simulink model "object_os"  (Simulink 8.7)
settings: Solver=ode45  StartTime=0.0  StopTime=3  FixedStep=0.01  RelTol=1e-3
settings Model: Creator=Andrew  LastModifiedBy=Dima
settings DataIOCC: ExternalInput=[a]  SignalLoggingSaveFormat=ModelDataLogs  SignalLogging=off  DSMLogging=off
settings OptimizationCC: DefaultParameterBehavior=Inlined  ExpressionDepthLimit=2147483647
settings DebuggingCC: SolverPrmCheckMsg=warning  FcnCallInpInsideContextMsg=UseLocalSettings  StateNameClashWarn=warning
settings GRTTargetCC: CombineOutputUpdateFcns=off  GRTInterface=on

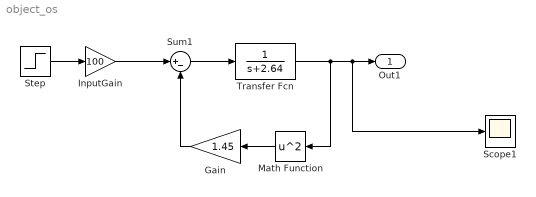
== system object_os ==
  Gain : Gain  Gain=1.45
  InputGain : Gain  Gain=100
  Math Function : Math  Operator=square  SaturateOnIntegerOverflow=on
  Scope1 : Scope
  Step : Step  Time=0.01  Before=1  After=0  SampleTime=0
  Sum1 : Sum  Inputs=|+-
  Transfer Fcn : TransferFcn  Denominator=[1 2.64]
  Out1 : Outport
  wires:
  Transfer Fcn/1 -> Math Function/1, Scope1/1, Out1/1
  Sum1/1 -> Transfer Fcn/1
  Math Function/1 -> Gain/1
  Gain/1 -> Sum1/2
  InputGain/1 -> Sum1/1
  Step/1 -> InputGain/1
